simulink model "SingleTankPIDControl_sim"  (R2021a)
settings: Solver=FixedStepAuto  StartTime=0.0  StopTime=40  FixedStep=0.1  RelTol=1e-3
InitFcn:
  | clearvars;
  | load('singletank_parameters.mat')
StopFcn:
  | plot_results
values from neighbouring files (symbols this model uses):
  params_single =     [singletank_parameters.mat]
libraries: simulink x1
settings Model: Creator=ksto036  LastModifiedBy=bl4ck
settings SolverCC: AlgebraicLoopSolver=TrustRegion
settings DataIOCC: SaveOutput=off  SignalLogging=off  DSMLogging=off  SaveTime=off  ReturnWorkspaceOutputs=off
settings DebuggingCC: SFMachineParentedDataDiag=warning

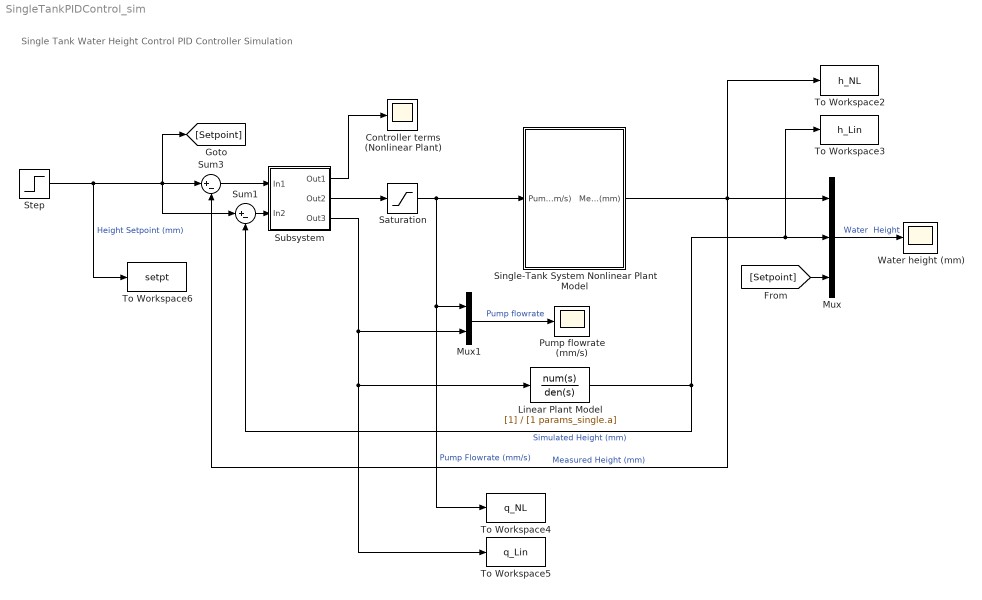
== system SingleTankPIDControl_sim ==
  note: Single Tank Water Height Control
      | PID Controller
      | Simulation
  " Single-Tank System Nonlinear Plant Model" : Subsystem
      mask Display: image('$imagefile'); % Use "Edit Image" on toolstrip to change.
  Controller terms (Nonlinear Plant) : Scope
  Linear Plant Model : TransferFcn  Denominator=[1 params_single.a]
  Mux : Mux  Inputs=3
  Mux1 : Mux  Inputs=2
  Pump flowrate (mm/s) : Scope
  Saturation : Saturate  UpperLimit=params_single.Qlimit  LowerLimit=0  LinearizeAsGain=off
  Step : Step  Time=0  After=150  SampleTime=0
  Subsystem : Subsystem  mask(PID Controller){P=0.35, I=0.01, D=0, I_limit=inf}
      mask prompts: P "Proportional"; I "Integral"; D "Derivative"; I_limit "Intergral term saturation limit (mm/s)"
      mask help:
      | Enter expressions for proportional, integral, and derivative terms.
      | P+I/s+Ds
      mask Help: This block implements a PID controller where parameters are entered for the Proportional, Integral and Derivative terms. Unmask this block to see how it works. The derivative term is implemented using a true derivative block. Allows the same gains to be used by two systems.
      mask Display: disp('PID')
  Sum1 : Sum  Inputs=|+-
  Sum3 : Sum  Inputs=|+-
  To Workspace2 : ToWorkspace  VariableName=h_NL  SaveFormat=Structure With Time  SampleTime=-1
  To Workspace3 : ToWorkspace  VariableName=h_Lin  SaveFormat=Structure With Time  SampleTime=-1
  To Workspace4 : ToWorkspace  VariableName=q_NL  SaveFormat=Structure With Time  SampleTime=-1
  To Workspace5 : ToWorkspace  VariableName=q_Lin  SaveFormat=Structure With Time  SampleTime=-1
  To Workspace6 : ToWorkspace  VariableName=setpt  SaveFormat=Structure With Time  SampleTime=-1
  Water height (mm) : Scope
  wires:
  Step/1 -> [Setpoint], Sum3/1, Sum1/1, To Workspace6/1  "Height Setpoint (mm)"
  Linear Plant Model/1 -> Sum1/2, Mux/2, To Workspace3/1  "Simulated Height (mm)"
  Mux/1 -> Water height (mm)/1  "Water  Height"
  Sum3/1 -> Subsystem/1(In1)
  Mux1/1 -> Pump flowrate (mm/s)/1  "Pump flowrate"
  Sum1/1 -> Subsystem/2(In2)
  Saturation/1 -> " Single-Tank System Nonlinear Plant Model"/1(Pump Flowrate (mm/s)), Mux1/1, To Workspace4/1  "Pump Flowrate (mm/s)"
  " Single-Tank System Nonlinear Plant Model"/1(Measured Height (mm)) -> To Workspace2/1, Mux/1, Sum3/2  "Measured Height (mm)"
  [Setpoint] -> Mux/3
  Subsystem/3(Out3) -> To Workspace5/1, Linear Plant Model/1, Mux1/2
  Subsystem/2(Out2) -> Saturation/1
  Subsystem/1(Out1) -> Controller terms (Nonlinear Plant)/1

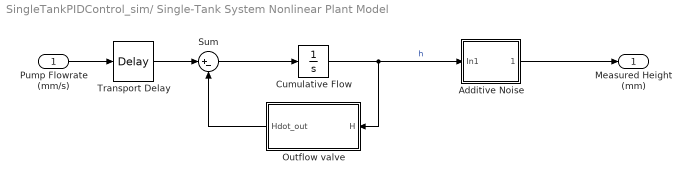
== system SingleTankPIDControl_sim/ Single-Tank System Nonlinear Plant Model ==
  Pump Flowrate (mm/s) : Inport
  Additive Noise : Subsystem
  Cumulative Flow : Integrator  LimitOutput=on  UpperSaturationLimit=params_single.Hlimit  LowerSaturationLimit=0
  Outflow valve : Subsystem
  Sum : Sum  Inputs=|+-
  Transport Delay : TransportDelay
  Measured Height (mm) : Outport  VectorParamsAs1DForOutWhenUnconnected=off
  wires:
  Sum/1 -> Cumulative Flow/1
  Cumulative Flow/1 -> Additive Noise/1(In1), Outflow valve/1(H)  "h"
  Outflow valve/1(Hdot_out) -> Sum/2
  Additive Noise/1(Measured Height (mm)) -> Measured Height (mm)/1
  Pump Flowrate (mm/s)/1 -> Transport Delay/1
  Transport Delay/1 -> Sum/1

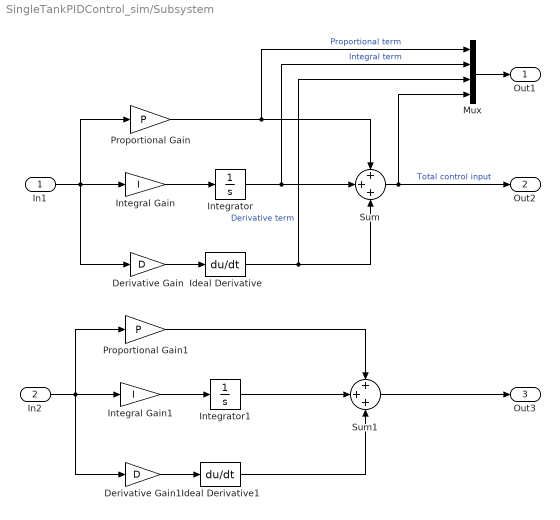
== system SingleTankPIDControl_sim/Subsystem ==
  In1 : Inport
  In2 : Inport  Port=2
  Derivative Gain : Gain  Gain=D  SaturateOnIntegerOverflow=on  OutDataTypeStr=Inherit: Same as input  ParamDataTypeStr=Inherit: Same as input
  Derivative Gain1 : Gain  Gain=D  SaturateOnIntegerOverflow=on  OutDataTypeStr=Inherit: Same as input  ParamDataTypeStr=Inherit: Same as input
  Ideal Derivative : Derivative
  Ideal Derivative1 : Derivative
  Integral Gain : Gain  Gain=I  SaturateOnIntegerOverflow=on  OutDataTypeStr=Inherit: Same as input  ParamDataTypeStr=Inherit: Same as input
  Integral Gain1 : Gain  Gain=I  SaturateOnIntegerOverflow=on  OutDataTypeStr=Inherit: Same as input  ParamDataTypeStr=Inherit: Same as input
  Integrator : Integrator  LimitOutput=on  UpperSaturationLimit=I_limit  LowerSaturationLimit=0
  Integrator1 : Integrator
  Mux : Mux
  Proportional Gain : Gain  Gain=P  SaturateOnIntegerOverflow=on  OutDataTypeStr=Inherit: Same as input  ParamDataTypeStr=Inherit: Same as input
  Proportional Gain1 : Gain  Gain=P  SaturateOnIntegerOverflow=on  OutDataTypeStr=Inherit: Same as input  ParamDataTypeStr=Inherit: Same as input
  Sum : Sum  Inputs=+++  InputSameDT=on  SaturateOnIntegerOverflow=on  OutDataTypeStr=Inherit: Same as first input
  Sum1 : Sum  Inputs=+++  InputSameDT=on  SaturateOnIntegerOverflow=on  OutDataTypeStr=Inherit: Same as first input
  Out1 : Outport
  Out2 : Outport  Port=2
  Out3 : Outport  Port=3
  wires:
  Integrator/1 -> Mux/2, Sum/2  "Integral term"
  Integral Gain/1 -> Integrator/1
  Proportional Gain/1 -> Mux/1, Sum/1  "Proportional term"
  Derivative Gain1/1 -> Ideal Derivative1/1
  In1/1 -> Derivative Gain/1, Integral Gain/1, Proportional Gain/1
  Ideal Derivative/1 -> Mux/3, Sum/3  "Derivative term"
  Derivative Gain/1 -> Ideal Derivative/1
  In2/1 -> Derivative Gain1/1, Integral Gain1/1, Proportional Gain1/1
  Sum1/1 -> Out3/1
  Integral Gain1/1 -> Integrator1/1
  Proportional Gain1/1 -> Sum1/1
  Sum/1 -> Out2/1, Mux/4  "Total control input"
  Ideal Derivative1/1 -> Sum1/3
  Integrator1/1 -> Sum1/2
  Mux/1 -> Out1/1

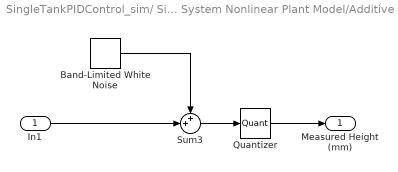
== system SingleTankPIDControl_sim/ Single-Tank System Nonlinear Plant Model/Additive Noise ==
  In1 : Inport
  Band-Limited White Noise : simulink/Sources/Band-Limited White Noise  Cov=[0.01]  Ts=0.1  seed=[23341]
  Quantizer : Quantizer  QuantizationInterval=0.2
  Sum3 : Sum  Inputs=++|  SaturateOnIntegerOverflow=on
  Measured Height (mm) : Outport  VectorParamsAs1DForOutWhenUnconnected=off
  wires:
  In1/1 -> Sum3/2
  Sum3/1 -> Quantizer/1
  Band-Limited White Noise/1 -> Sum3/1
  Quantizer/1 -> Measured Height (mm)/1

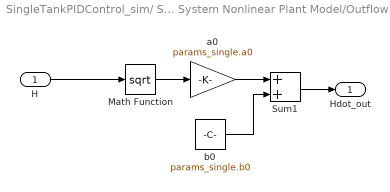
== system SingleTankPIDControl_sim/ Single-Tank System Nonlinear Plant Model/Outflow valve ==
  H : Inport
  Math Function : Math  Operator=sqrt  SignedPower=on  SaturateOnIntegerOverflow=on
  Sum1 : Sum  SaturateOnIntegerOverflow=on
  a0 : Gain  Gain=params_single.a0  SaturateOnIntegerOverflow=on  OutDataTypeStr=Inherit: Same as input  ParamDataTypeStr=Inherit: Same as input
  b0 : Constant  Value=params_single.b0
  Hdot_out : Outport  VectorParamsAs1DForOutWhenUnconnected=off
  wires:
  b0/1 -> Sum1/2
  Sum1/1 -> Hdot_out/1
  H/1 -> Math Function/1
  a0/1 -> Sum1/1
  Math Function/1 -> a0/1
